simulink model "Appl_HeatAdj_CtrlModel"  (R2018b)
settings: configuration reference "CodeConfig_10_ms" (kept outside this file)
undefined symbols (not defined in the file): CAL_LEVEL3_TIMEOUT, CAL_SW_20min_TIMEOUT, D_1stLevel_36, D_2ndLevel_39, D_3rdLevel_45, D_3rdLevel_48, D_DRVHEAT_PID_D, D_DRVHEAT_PID_I, D_DRVHEAT_PID_P, D_HEAT_HEAT_DEF, D_SwsLevel_Temp, FALSE, TRUE
libraries: DareLib x111, simulink x1
(part 5 of 6)

== stateflow chart Appl_HeatAdj_CtrlModel/LogicCtrl/LocalAdjustCtrl/OutputDeal/HeatOutFunction2/HeatOut ==
  state PwmCnt = PidGetPwm(CurrentTemp,SetTemp) [function]
  state Controll [parallel]
    settings: executionOrder=1
    state AllOut
      en:
      du:
      HeatOutGpio = ON;
      HeatOutPwmCnt =100;
      TimeCnt = 0;
    state None
      en:
      du:
      HeatOutGpio = OFF;
      HeatOutPwmCnt = 0;
      TimeCnt = 0;
    state PwmOut
      en:
      HeatOutPwmCnt = PidGetPwm(CurrentTemp,SetTemp);
      (default) -> (junction 11)
      PwmOut -> (junction 11) [order 1]
      (junction 11) -> (junction 12) [order 1] : /* 100计数 */
          | [TimeCnt <= 100]
      (junction 11) -> (junction 15) [order 2] : /* 计算pid 算pwm */
          | {TimeCnt = 0;
          | HeatOutPwmCnt = PidGetPwm(CurrentTemp,SetTemp);}
      (junction 12) -> (junction 13) : {TimeCnt += 1;}
      (junction 13) -> (junction 14) [order 1] : [TimeCnt <= HeatOutPwmCnt]
      (junction 13) -> (junction 16) [order 2] : /* 引脚拉低 */
          | {HeatOutGpio = OFF;}
      (junction 14) -> (junction 17) : /* 引脚拉高 */
          | {HeatOutGpio = ON;}
      (junction 16) -> (junction 15)
      (junction 17) -> (junction 16)
      (junction 15) -> (junction 18)
    (default) -> None
    None -> AllOut [order 1] : /* 加热误差在3度 全开 */
        | [enHeatLvlSts.EN_HEAT_LVL_OFF < HeatLvl ...
        | && SetTemp > CurrentTemp ...
        | && (SetTemp - CurrentTemp) >= D_HEAT_HEAT_DEF]
    AllOut -> None [order 1] : /*全开 进 关 */
        | [SetTemp <= CurrentTemp ...
        | || enHeatLvlSts.EN_HEAT_LVL_OFF == HeatLvl]
    PwmOut -> None [order 1] : /* PID 进 关 */
        | [SetTemp <= CurrentTemp ...
        | || enHeatLvlSts.EN_HEAT_LVL_OFF == HeatLvl]
    None -> PwmOut [order 2] : /* 关 进 PID */
        | [enHeatLvlSts.EN_HEAT_LVL_OFF < HeatLvl ...
        | && SetTemp > CurrentTemp ...
        | && (SetTemp - CurrentTemp) < D_HEAT_HEAT_DEF]
    PwmOut -> AllOut [order 2] : /* 加热误差在3度 全开 */
        | [enHeatLvlSts.EN_HEAT_LVL_OFF < HeatLvl ...
        | && SetTemp > CurrentTemp ...
        | && (SetTemp - CurrentTemp) >= D_HEAT_HEAT_DEF]
    AllOut -> PwmOut [order 2] : /* 全开 进PID */
        | [enHeatLvlSts.EN_HEAT_LVL_OFF < HeatLvl ...
        | && SetTemp > CurrentTemp ...
        | && (SetTemp - CurrentTemp) < D_HEAT_HEAT_DEF]
  state count [parallel]
    settings: executionOrder=2
    (default) -> (junction 47)
    count -> (junction 47)
    (junction 47) -> (junction 50) [order 1] : /*方向盘加热开启且加热温度≥目标温度*/
        | [enHeatLvlSts.EN_HEAT_LVL_OFF < HeatLvl ...
        | && CurrentTemp >= (SetTemp - 20)]
    (junction 47) -> (junction 52) [order 2] : {Sw20minTimer = D_HAL_GET_CUR_MS_TS();}
    (junction 50) -> (junction 54)
    (junction 54) -> (junction 58) [order 1] : [TimeDiffTs(Sw20minTimer,D_HAL_GET_CUR_MS_TS()) < MaxTime]
    (junction 54) -> (junction 62) [order 2] : {SwTimeoutFlag = TRUE;}
    (junction 58) -> (junction 60) : {SwTimeoutFlag = FALSE;}
    (junction 62) -> (junction 52)
    (junction 60) -> (junction 62)
    (junction 52) -> (junction 66)
    (junction 66) -> (junction 82) [order 1] : [enHeatLvlSts.EN_HEAT_LVL_OFF == HeatLvl]
    (junction 66) -> (junction 87) [order 2]
    (junction 82) -> (junction 84) : {SwTimeoutFlag = FALSE;}
    (junction 84) -> (junction 87)
    (junction 87) -> (junction 92)
  state Ts = D_HAL_GET_CUR_MS_TS [function]
  state OutTs = TimeDiffTs(lastTs,Ts) [function]
  state count1 [parallel] [commented out]
    (default) -> (junction 103) [commented out]
    count1 -> (junction 103) [commented out]
    (junction 103) -> (junction 105) [commented out] : /*方向盘加热开启且加热温度≥目标温度*/
        | [enHeatLvlSts.EN_HEAT_LVL_OFF < HeatLvl ...
        | && CurrentTemp >= (SetTemp - 20)]
    (junction 103) -> (junction 111) [commented out]
    (junction 105) -> (junction 106) [commented out]
    (junction 106) -> (junction 108) [commented out] : [MaxTime > Sw20minTimer]
    (junction 106) -> (junction 107) [commented out] : {Sw20minTimer = MaxTime;
        | SwTimeoutFlag = TRUE;}
    (junction 108) -> (junction 113) [commented out] : {Sw20minTimer ++;
        | SwTimeoutFlag = FALSE;}
    (junction 107) -> (junction 111) [commented out]
    (junction 113) -> (junction 107) [commented out]
    (junction 111) -> (junction 114) [commented out]
    (junction 114) -> (junction 118) [commented out] : [enHeatLvlSts.EN_HEAT_LVL_OFF == HeatLvl]
    (junction 114) -> (junction 120) [commented out]
    (junction 118) -> (junction 102) [commented out] : {Sw20minTimer = 0;
        | SwTimeoutFlag = FALSE;}
    (junction 102) -> (junction 120) [commented out]
    (junction 120) -> (junction 101) [commented out]
  data: CurrentTemp function_input; PwmCnt function_output; SetTemp function_input; Ts function_output; lastTs function_input; Ts function_input; OutTs function_output; CurrentTemp input uint16; HeatLvl input Enum: enHeatLvlSts; SetTemp input uint16; HeatOutGpio output uint8; TimeCnt local uint8; OFF parameter; ON parameter; D_HEAT_HEAT_DEF parameter; HeatOutPwmCnt output uint8; TRUE parameter; FALSE parameter; SwTimeoutFlag output uint8 =0; Sw20minTimer output uint32; MaxTime input

== stateflow chart Appl_HeatAdj_CtrlModel/LogicCtrl/LocalAdjustCtrl/OutputDeal/HeatOutFunction2/HeatOut/PidGetPwm/Pid  ==
  (default) -> (junction 14)
  (junction 14) -> (junction 16) : /* 局部初始化 */
      | {Error = 0;
      | dError = 0;}
  (junction 16) -> (junction 20) : /* PID 计算 */
      | {Error = SetTemp - CurrentTemp;
      | SumError += Error;
      | dError = Error - LastError;
      | LastError = Error;
      | PwmCnt = (D_DRVHEAT_PID_P * Error)  + (D_DRVHEAT_PID_I *SumError) + (D_DRVHEAT_PID_D *  dError);}
  (junction 20) -> (junction 29) [order 1] : [PwmCnt > 100]
  (junction 20) -> (junction 27) [order 2]
  (junction 29) -> (junction 31) : {PwmCnt = 100;}
  (junction 31) -> (junction 27)
  (junction 27) -> (junction 34)
  data: dError local uint32; Error local uint32; CurrentTemp input uint16; SetTemp input uint16; PwmCnt output uint16; SumError local uint32; LastError local uint32; D_DRVHEAT_PID_P parameter; D_DRVHEAT_PID_I parameter; D_DRVHEAT_PID_D parameter

== stateflow chart Appl_HeatAdj_CtrlModel/LogicCtrl/LocalAdjustCtrl/LimitDeal/TimeoutFunction/Timeout ==
  state Ts = D_HAL_GET_CUR_MS_TS [function]
  state OutTs = TimeDiffTs(lastTs,Ts) [function]
  state TimeCountStatus
    state TimeoutSts
      en:
      Level = enHeatLvlSts.EN_HEAT_LVL_OFF;
      du:
      Level = enHeatLvlSts.EN_HEAT_LVL_OFF;
      ex:
      Timer = 0;
    state Init
      en:
      Level = InLevel;
      Timer = D_HAL_GET_CUR_MS_TS();
      du:
      Level = InLevel;
      ex:
      Timer = D_HAL_GET_CUR_MS_TS();
    (default) -> Init
    Init -> TimeoutSts [order 1] : [TimeDiffTs(Timer,D_HAL_GET_CUR_MS_TS()) >= MaxTime]
        | /TimeoutFlag = TRUE;
    TimeoutSts -> Init : [hasChangedFrom(InLevel,enHeatLvlSts.EN_HEAT_LVL_OFF)]
    Init -> Init [order 2] : [hasChangedFrom(InLevel,enHeatLvlSts.EN_HEAT_LVL_OFF)]
  state Default
    en:
    Level = InLevel;
    du:
    Level = InLevel;
  (default) -> Default
  Default -> TimeCountStatus : /*有超时配置
      | && 启动加热&&有时间值 */
      | [TRUE == TimeoutPrm ...
      | && enHeatLvlSts.EN_HEAT_LVL_OFF != InLevel ...
      | && 0 != MaxTime]
  TimeCountStatus -> Default : /*无超时配置*/
      | [TRUE != TimeoutPrm || 0 == MaxTime]
      | /TimeoutFlag = FALSE;
  data: Ts function_output; lastTs function_input; Ts function_input; OutTs function_output; TimeoutPrm input uint8; TimeoutFlag output uint8; FALSE parameter; TRUE parameter; InLevel input Enum: enHeatLvlSts; MaxTime input uint32; Timer local uint32; Level output Enum: enHeatLvlSts

== stateflow chart Appl_HeatAdj_CtrlModel/LogicCtrl/LocalAdjustCtrl/LimitDeal/TimeoutFunction/Timeout/TimeDiffTs/Chart ==
  (default) -> (junction 3)
  (junction 3) -> (junction 5)
  (junction 5) -> (junction 7) [order 1] : /* 入参比当前大 */
      | [lastTs > Ts]
  (junction 5) -> (junction 13) [order 2] : {OutTs = Ts - lastTs;}
  (junction 7) -> (junction 11) : {OutTs = 0xFFFFFFFF - lastTs + Ts +1;}
  (junction 11) -> (junction 13)
  (junction 13) -> (junction 17)
  data: lastTs input uint32; Ts input uint32; OutTs output uint32

== stateflow chart Appl_HeatAdj_CtrlModel/LogicCtrl/LocalAdjustCtrl/HeatLevelDeal/LevelAquireFunction2/LevelAquireFunction ==
  state LevelAquire
    (default) -> (junction 103)
    LevelAquire -> (junction 103)
    (junction 103) -> (junction 105) [order 1] : /*加热功能禁能
        | || 通用前置条件不满足)*/
        | [enHeatStopReason.EN_HEAT_STOP_R_NONE != DisableSts ...
        | || FALSE == EnableCfg ...
        | || TRUE != ComPCFlag]
    (junction 103) -> (junction 102) [order 2] : {StopFlag = FALSE;}
    (junction 105) -> (junction 104) : {Level = enHeatLvlSts.EN_HEAT_LVL_OFF;
        | StopFlag = TRUE;}
    (junction 104) -> (junction 102)
    (junction 102) -> (junction 111)
    (junction 111) -> (junction 21) [order 1] : [FALSE == StopFlag]
    (junction 21) -> (junction 23) [order 1] : [enProjectType.EN_PROJECT_P20 == CarTypeCfg]
    (junction 111) -> (junction 114) [order 2] : {Level = enHeatLvlSts.EN_HEAT_LVL_OFF;}
    (junction 21) -> (junction 48) [order 2]
    (junction 23) -> (junction 85)
    (junction 85) -> (junction 87) [order 1] : /* open 信号 且为HMI控制*/
        | [5 == CAN_Message && Type == FALSE]
    (junction 85) -> (junction 25) [order 2]
    (junction 87) -> (junction 89) : {Level = CanLvl + 1;}
    (junction 25) -> (junction 27) [order 1] : [4 == CAN_Message]
    (junction 25) -> (junction 29) [order 2] : {TempMsg = CAN_Message + 1;}
    (junction 27) -> (junction 57) : {Level = enHeatLvlSts.EN_HEAT_LVL_OFF;}
    (junction 48) -> (junction 50) [order 1] : [1 != CAN_Message]
    (junction 48) -> (junction 55) [order 2] : {Level = enHeatLvlSts.EN_HEAT_LVL_OFF;}
    (junction 50) -> (junction 52) : {TempMsg = CAN_Message;}
    (junction 52) -> (junction 29)
    (junction 29) -> (junction 32) [order 1] : [1 < TempMsg && 5 > TempMsg]
    (junction 29) -> (junction 36) [order 2] : {Level = 0xFF;}
    (junction 32) -> (junction 34)
    (junction 34) -> (junction 38) [order 1] : [2 == TempMsg]
    (junction 34) -> (junction 40) [order 2]
    (junction 38) -> (junction 59) : {Level = enHeatLvlSts.EN_HEAT_LVL_1;}
    (junction 40) -> (junction 42) [order 1] : [3 == TempMsg]
    (junction 40) -> (junction 46) [order 2] : {Level = enHeatLvlSts.EN_HEAT_LVL_3;}
    (junction 42) -> (junction 44) : {Level = enHeatLvlSts.EN_HEAT_LVL_2;}
    (junction 55) -> (junction 114)
    (junction 36) -> (junction 55)
    (junction 46) -> (junction 36)
    (junction 44) -> (junction 46)
    (junction 59) -> (junction 44)
    (junction 57) -> (junction 59)
    (junction 89) -> (junction 57)
    (junction 114) -> (junction 75)
  data: EnableCfg input uint8; CarTypeCfg input Enum: enProjectType; CAN_Message input uint8; DisableSts input Enum: enHeatStopReason; Level output uint8; TempMsg local uint8; TRUE parameter; FALSE parameter; ComPCFlag input; CanLvl input uint8; Type input; CurLvl input; StopFlag local boolean

== stateflow chart Appl_HeatAdj_CtrlModel/UpDataInputInfo/InputSignalProcess/HeatMessage/HeatMessage ==
  state [OutMsgHMI,OutMsgTbox,MixConflictFlg] = MsgConflictFunction2(CarTypeCfg,HMI_Message,Tbox_Message,VentValidFlag) [function]
  state [OutMsgHMI,OutMsgTbox,MixConflictFlg] = MsgConflictFunction1(CarTypeCfg,HMI_Message,Tbox_Message,VentValidFlag) [function]
  state [OutMsgHMI,OutMsgTbox,MixConflictFlg] = MsgConflictFunction(CarTypeCfg,HMI_Message,Tbox_Message,VentValidFlag) [function]
  state Message
    du:
    [DriverHMI_Message,DriverTbox_Message,Driver_MixConflicFlg] = MsgConflictFunction(HeatAdj_CarType,HeatAdj_DriverHMI_Message,HeatAdj_DriverTbox_Message,DriverVentilateValid);
    [PassengerHMI_Message,PassengerTbox_Message,Passenger_MixConflicFlg] = MsgConflictFunction1(HeatAdj_CarType,HeatAdj_PassengerHMI_Message,HeatAdj_PassengerTbox_Message,PassengerVentilateValid);
    [ThirdHMI_Message,ThirdTbox_Message,Third_MixConflicFlg] = MsgConflictFunction2(HeatAdj_CarType,HeatAdj_ThirdHMI_Message,HeatAdj_ThirdTbox_Message,ThirdVentilateValid);
  (default) -> Message
  data: CarTypeCfg function_input; HMI_Message function_input uint8; Tbox_Message function_input uint8; VentValidFlag function_input; OutMsgHMI function_output; OutMsgTbox function_output; MixConflictFlg function_output; CarTypeCfg function_input; HMI_Message function_input uint8; Tbox_Message function_input uint8; VentValidFlag function_input; OutMsgHMI function_output; OutMsgTbox function_output; MixConflictFlg function_output; CarTypeCfg function_input; HMI_Message function_input uint8; Tbox_Message function_input uint8; VentValidFlag function_input; OutMsgHMI function_output; OutMsgTbox function_output; MixConflictFlg function_output; DriverHMI_Message output uint8; DriverTbox_Message output uint8; PassengerHMI_Message output uint8; HeatAdj_DriverHMI_Message input; HeatAdj_DriverTbox_Message input; HeatAdj_PassengerHMI_Message input; HeatAdj_PassengerTbox_Message input; HeatAdj_ThirdHMI_Message input; HeatAdj_ThirdTbox_Message input; DriverVentilateValid input; PassengerVentilateValid input; ThirdVentilateValid input; PassengerTbox_Message output uint8; ThirdHMI_Message output uint8; ThirdTbox_Message output uint8; HeatAdj_CarType input; Driver_MixConflicFlg output uint8; Passenger_MixConflicFlg output uint8; Third_MixConflicFlg output uint8

== stateflow chart Appl_HeatAdj_CtrlModel/UpDataInputInfo/InputSignalProcess/HeatMessage/HeatMessage/MsgConflictFunction/Function ==
  state HMI_MessageDeal [parallel]
    settings: executionOrder=1
    state Default
      en:
      HMI_Flag = FALSE;
    state Valid
      en:
      HMI_Flag = TRUE;
    (default) -> HMI_MessageDeal.Default
    HMI_MessageDeal.Default -> HMI_MessageDeal.Valid : /*HMI加热报文有效0x0:Inactive；0x1:Level 1；1档;0x2:Level 2；2档;0x3:Level 3；3档；0x4:OFF: 0x05 OPEN*/
        | [enHeatLvlSts.EN_HEAT_LVL_1 == HMI_Message ...
        | || enHeatLvlSts.EN_HEAT_LVL_2 == HMI_Message ...
        | || enHeatLvlSts.EN_HEAT_LVL_3 == HMI_Message ...
        | || 4 == HMI_Message || 5 == HMI_Message]
    HMI_MessageDeal.Valid -> HMI_MessageDeal.Default : /*HMI加热报文无效，20240507NXM增加关闭4*/
        | [enHeatLvlSts.EN_HEAT_LVL_1 != HMI_Message ...
        | && enHeatLvlSts.EN_HEAT_LVL_2 != HMI_Message ...
        | && enHeatLvlSts.EN_HEAT_LVL_3 != HMI_Message ...
        | && 4 != HMI_Message && 5 != HMI_Message]
  state Tbox_MessageDeal [parallel]
    settings: executionOrder=2
    state Default
      en:
      Tbox_Flag = FALSE;
    state Valid
      en:
      Tbox_Flag = TRUE;
    (default) -> Tbox_MessageDeal.Default
    Tbox_MessageDeal.Default -> Tbox_MessageDeal.Valid : /*Tbox加热报文有效0x0:No Request；0x1:Heat_1；0x2:Heat_2；0x3:Heat_3；0x4:Close*/
        | [enHeatLvlSts.EN_HEAT_LVL_1 == Tbox_Message ...
        | || enHeatLvlSts.EN_HEAT_LVL_2 == Tbox_Message ...
        | || enHeatLvlSts.EN_HEAT_LVL_3 == Tbox_Message ...
        | || 4 == Tbox_Message]
    Tbox_MessageDeal.Valid -> Tbox_MessageDeal.Default : /*Tbox加热报文无效，20240507NXM增加关闭4*/
        | [enHeatLvlSts.EN_HEAT_LVL_1 != Tbox_Message ...
        | && enHeatLvlSts.EN_HEAT_LVL_2 != Tbox_Message ...
        | && enHeatLvlSts.EN_HEAT_LVL_3 != Tbox_Message ...
        | && 4 != Tbox_Message]
  state MessageConflictDeal [parallel]
    settings: executionOrder=3
    state Default
      en,du:
      OutMsgHMI = HMI_Message;
      OutMsgTbox = Tbox_Message;
      MixConflictFlg = FALSE;
    state VentilateConflict
      en:
      OutMsgHMI = 0;
      OutMsgTbox = 0;
      MixConflictFlg = TRUE;
    state HeatConflict
      en:
      OutMsgHMI = 0;
      OutMsgTbox = 0;
      MixConflictFlg = FALSE;
    (default) -> MessageConflictDeal.Default
    MessageConflictDeal.Default -> VentilateConflict [order 2] : /*通风加热报文同时有效 不包含关闭 */
        | [FALSE != VentValidFlag ...
        | && ((FALSE != HMI_Flag && 4 != HMI_Message)...
        | || (FALSE != Tbox_Flag && 4 != Tbox_Message))]
    VentilateConflict -> MessageConflictDeal.Default [order 2] : /*通风加热报文不同时有效或关闭，20240507NXM修改跳转顺序*/
        | [FALSE == VentValidFlag ...
        | || 4 == HMI_Message ...
        | || 4 == Tbox_Message]
    MessageConflictDeal.Default -> HeatConflict [order 1] : /*P20车型HMI、TBOX加热报文同时有效*/
        | [enProjectType.EN_PROJECT_P20 == CarTypeCfg ...
        | && FALSE != HMI_Flag ...
        | && FALSE != Tbox_Flag]
    HeatConflict -> MessageConflictDeal.Default [order 2] : /*非P20车型||P20车型加热报文不同时有效，20240507NXM*/
        | [enProjectType.EN_PROJECT_P20 != CarTypeCfg ...
        | || (enProjectType.EN_PROJECT_P20 == CarTypeCfg ...
        | && (FALSE == HMI_Flag || FALSE == Tbox_Flag))]
    VentilateConflict -> HeatConflict [order 1] : /*P20车型HMI、TBOX加热报文同时有效*/
        | [enProjectType.EN_PROJECT_P20 == CarTypeCfg ...
        | && FALSE != HMI_Flag ...
        | && FALSE != Tbox_Flag ...
        | && FALSE == VentValidFlag]
    HeatConflict -> VentilateConflict [order 1] : /*通风加热报文同时有效，20240507NXM*/
        | [FALSE != VentValidFlag ...
        | && (FALSE != HMI_Flag ...
        | || FALSE != Tbox_Flag)]
  data: CarTypeCfg input uint8; HMI_Message input; Tbox_Message input; VentValidFlag input uint8; FALSE parameter; OutMsgHMI output uint8; OutMsgTbox output uint8; HMI_Flag local uint8; Tbox_Flag local uint8; TRUE parameter; MixConflictFlg output uint8

== stateflow chart Appl_HeatAdj_CtrlModel/UpDataInputInfo/InputSignalProcess/CommonPreconditionDeal/Deal ==
  state Default
    en:
    ComPCSatisfiedFlag = FALSE;
  state ValidSts
    en:
    ComPCSatisfiedFlag = TRUE;
  (default) -> Default
  Default -> ValidSts : /*非OFF电 && DCDC开关状态为使能
      | && 正常电压模式下
      | && (发动机运行中 || 整车运行状态满足)*/
      | [enPowerModeSts.EN_OFF != HeatAdj_PowerMode ...
      | && TRUE == DCDC_SwitchEnable ...
      | && enFinalPowerMode.EN_NORMAL_VOLT == HeatAdj_VoltMode ...
      | && (TRUE == EngineRunningFlag || TRUE == VehicleRunFlag)]
  ValidSts -> Default : /*OFF电 || DCDC开关状态为非使能 || 非正常电压
      | || (发动机不在运行中 && 整车运行状态不满足)*/
      | [enPowerModeSts.EN_OFF == HeatAdj_PowerMode ...
      | || TRUE != DCDC_SwitchEnable ...
      | || enFinalPowerMode.EN_NORMAL_VOLT != HeatAdj_VoltMode ...
      | || (TRUE != EngineRunningFlag && TRUE != VehicleRunFlag)]
  data: HeatAdj_PowerMode input; DCDC_SwitchEnable input; EngineRunningFlag input; VehicleRunFlag input; ComPCSatisfiedFlag output uint8; TRUE parameter; FALSE parameter; HeatAdj_VoltMode input

== stateflow chart Appl_HeatAdj_CtrlModel/LogicCtrl/LocalAdjustCtrl/HeatLevelDeal/LevelAquireFunction4/LevelAquireFunction ==
  state LevelAquire
    (default) -> (junction 103)
    LevelAquire -> (junction 103)
    (junction 103) -> (junction 105) [order 1] : /*加热功能禁能
        | || 通用前置条件不满足)*/
        | [enHeatStopReason.EN_HEAT_STOP_R_NONE != DisableSts ...
        | || FALSE == EnableCfg ...
        | || TRUE != ComPCFlag]
    (junction 103) -> (junction 102) [order 2] : {StopFlag = FALSE;}
    (junction 105) -> (junction 104) : {Level = enHeatLvlSts.EN_HEAT_LVL_OFF;
        | StopFlag = TRUE;}
    (junction 104) -> (junction 102)
    (junction 102) -> (junction 111)
    (junction 111) -> (junction 21) [order 1] : [FALSE == StopFlag]
    (junction 21) -> (junction 23) [order 1] : [enProjectType.EN_PROJECT_P20 == CarTypeCfg]
    (junction 111) -> (junction 114) [order 2] : {Level = enHeatLvlSts.EN_HEAT_LVL_OFF;}
    (junction 21) -> (junction 48) [order 2]
    (junction 23) -> (junction 85)
    (junction 85) -> (junction 87) [order 1] : /* open 信号 且为HMI控制*/
        | [5 == CAN_Message && Type == FALSE]
    (junction 85) -> (junction 25) [order 2]
    (junction 87) -> (junction 89) : {Level = CanLvl + 1;}
    (junction 25) -> (junction 27) [order 1] : [4 == CAN_Message]
    (junction 25) -> (junction 29) [order 2] : {TempMsg = CAN_Message + 1;}
    (junction 27) -> (junction 57) : {Level = enHeatLvlSts.EN_HEAT_LVL_OFF;}
    (junction 48) -> (junction 50) [order 1] : [1 != CAN_Message]
    (junction 48) -> (junction 55) [order 2] : {Level = enHeatLvlSts.EN_HEAT_LVL_OFF;}
    (junction 50) -> (junction 52) : {TempMsg = CAN_Message;}
    (junction 52) -> (junction 29)
    (junction 29) -> (junction 32) [order 1] : [1 < TempMsg && 5 > TempMsg]
    (junction 29) -> (junction 36) [order 2] : {Level = 0xFF;}
    (junction 32) -> (junction 34)
    (junction 34) -> (junction 38) [order 1] : [2 == TempMsg]
    (junction 34) -> (junction 40) [order 2]
    (junction 38) -> (junction 59) : {Level = enHeatLvlSts.EN_HEAT_LVL_1;}
    (junction 40) -> (junction 42) [order 1] : [3 == TempMsg]
    (junction 40) -> (junction 46) [order 2] : {Level = enHeatLvlSts.EN_HEAT_LVL_3;}
    (junction 42) -> (junction 44) : {Level = enHeatLvlSts.EN_HEAT_LVL_2;}
    (junction 55) -> (junction 114)
    (junction 36) -> (junction 55)
    (junction 46) -> (junction 36)
    (junction 44) -> (junction 46)
    (junction 59) -> (junction 44)
    (junction 57) -> (junction 59)
    (junction 89) -> (junction 57)
    (junction 114) -> (junction 75)
  data: EnableCfg input uint8; CarTypeCfg input Enum: enProjectType; CAN_Message input uint8; DisableSts input Enum: enHeatStopReason; Level output uint8; TempMsg local uint8; TRUE parameter; FALSE parameter; ComPCFlag input; CanLvl input uint8; Type input; CurLvl input; StopFlag local boolean

== stateflow chart Appl_HeatAdj_CtrlModel/LogicCtrl/LocalAdjustCtrl/HeatLevelDeal/LevelAquireFunction/LevelAquireFunction ==
  state LevelAquire
    (default) -> (junction 103)
    LevelAquire -> (junction 103)
    (junction 103) -> (junction 105) [order 1] : /*加热功能禁能
        | || 通用前置条件不满足)*/
        | [enHeatStopReason.EN_HEAT_STOP_R_NONE != DisableSts ...
        | || FALSE == EnableCfg ...
        | || TRUE != ComPCFlag]
    (junction 103) -> (junction 102) [order 2] : {StopFlag = FALSE;}
    (junction 105) -> (junction 104) : {Level = enHeatLvlSts.EN_HEAT_LVL_OFF;
        | StopFlag = TRUE;}
    (junction 104) -> (junction 102)
    (junction 102) -> (junction 111)
    (junction 111) -> (junction 21) [order 1] : [FALSE == StopFlag]
    (junction 21) -> (junction 23) [order 1] : [enProjectType.EN_PROJECT_P20 == CarTypeCfg]
    (junction 111) -> (junction 114) [order 2] : {Level = enHeatLvlSts.EN_HEAT_LVL_OFF;}
    (junction 21) -> (junction 48) [order 2]
    (junction 23) -> (junction 85)
    (junction 85) -> (junction 87) [order 1] : /* open 信号 且为HMI控制*/
        | [5 == CAN_Message && Type == FALSE]
    (junction 85) -> (junction 25) [order 2]
    (junction 87) -> (junction 89) : {Level = CanLvl + 1;}
    (junction 25) -> (junction 27) [order 1] : [4 == CAN_Message]
    (junction 25) -> (junction 29) [order 2] : {TempMsg = CAN_Message + 1;}
    (junction 27) -> (junction 57) : {Level = enHeatLvlSts.EN_HEAT_LVL_OFF;}
    (junction 48) -> (junction 50) [order 1] : [1 != CAN_Message]
    (junction 48) -> (junction 55) [order 2] : {Level = enHeatLvlSts.EN_HEAT_LVL_OFF;}
    (junction 50) -> (junction 52) : {TempMsg = CAN_Message;}
    (junction 52) -> (junction 29)
    (junction 29) -> (junction 32) [order 1] : [1 < TempMsg && 5 > TempMsg]
    (junction 29) -> (junction 36) [order 2] : {Level = 0xFF;}
    (junction 32) -> (junction 34)
    (junction 34) -> (junction 38) [order 1] : [2 == TempMsg]
    (junction 34) -> (junction 40) [order 2]
    (junction 38) -> (junction 59) : {Level = enHeatLvlSts.EN_HEAT_LVL_1;}
    (junction 40) -> (junction 42) [order 1] : [3 == TempMsg]
    (junction 40) -> (junction 46) [order 2] : {Level = enHeatLvlSts.EN_HEAT_LVL_3;}
    (junction 42) -> (junction 44) : {Level = enHeatLvlSts.EN_HEAT_LVL_2;}
    (junction 55) -> (junction 114)
    (junction 36) -> (junction 55)
    (junction 46) -> (junction 36)
    (junction 44) -> (junction 46)
    (junction 59) -> (junction 44)
    (junction 57) -> (junction 59)
    (junction 89) -> (junction 57)
    (junction 114) -> (junction 75)
  data: EnableCfg input uint8; CarTypeCfg input Enum: enProjectType; CAN_Message input uint8; DisableSts input Enum: enHeatStopReason; Level output uint8; TempMsg local uint8; TRUE parameter; FALSE parameter; ComPCFlag input; CanLvl input uint8; Type input; CurLvl input; StopFlag local boolean

== stateflow chart Appl_HeatAdj_CtrlModel/LogicCtrl/LocalAdjustCtrl/HeatLevelDeal/LevelAquireFunction5/LevelAquireFunction ==
  state LevelAquire
    (default) -> (junction 103)
    LevelAquire -> (junction 103)
    (junction 103) -> (junction 105) [order 1] : /*加热功能禁能
        | || 通用前置条件不满足)*/
        | [enHeatStopReason.EN_HEAT_STOP_R_NONE != DisableSts ...
        | || FALSE == EnableCfg ...
        | || TRUE != ComPCFlag]
    (junction 103) -> (junction 102) [order 2] : {StopFlag = FALSE;}
    (junction 105) -> (junction 104) : {Level = enHeatLvlSts.EN_HEAT_LVL_OFF;
        | StopFlag = TRUE;}
    (junction 104) -> (junction 102)
    (junction 102) -> (junction 111)
    (junction 111) -> (junction 21) [order 1] : [FALSE == StopFlag]
    (junction 21) -> (junction 23) [order 1] : [enProjectType.EN_PROJECT_P20 == CarTypeCfg]
    (junction 111) -> (junction 114) [order 2] : {Level = enHeatLvlSts.EN_HEAT_LVL_OFF;}
    (junction 21) -> (junction 48) [order 2]
    (junction 23) -> (junction 85)
    (junction 85) -> (junction 87) [order 1] : /* open 信号 且为HMI控制*/
        | [5 == CAN_Message && Type == FALSE]
    (junction 85) -> (junction 25) [order 2]
    (junction 87) -> (junction 89) : {Level = CanLvl + 1;}
    (junction 25) -> (junction 27) [order 1] : [4 == CAN_Message]
    (junction 25) -> (junction 29) [order 2] : {TempMsg = CAN_Message + 1;}
    (junction 27) -> (junction 57) : {Level = enHeatLvlSts.EN_HEAT_LVL_OFF;}
    (junction 48) -> (junction 50) [order 1] : [1 != CAN_Message]
    (junction 48) -> (junction 55) [order 2] : {Level = enHeatLvlSts.EN_HEAT_LVL_OFF;}
    (junction 50) -> (junction 52) : {TempMsg = CAN_Message;}
    (junction 52) -> (junction 29)
    (junction 29) -> (junction 32) [order 1] : [1 < TempMsg && 5 > TempMsg]
    (junction 29) -> (junction 36) [order 2] : {Level = 0xFF;}
    (junction 32) -> (junction 34)
    (junction 34) -> (junction 38) [order 1] : [2 == TempMsg]
    (junction 34) -> (junction 40) [order 2]
    (junction 38) -> (junction 59) : {Level = enHeatLvlSts.EN_HEAT_LVL_1;}
    (junction 40) -> (junction 42) [order 1] : [3 == TempMsg]
    (junction 40) -> (junction 46) [order 2] : {Level = enHeatLvlSts.EN_HEAT_LVL_3;}
    (junction 42) -> (junction 44) : {Level = enHeatLvlSts.EN_HEAT_LVL_2;}
    (junction 55) -> (junction 114)
    (junction 36) -> (junction 55)
    (junction 46) -> (junction 36)
    (junction 44) -> (junction 46)
    (junction 59) -> (junction 44)
    (junction 57) -> (junction 59)
    (junction 89) -> (junction 57)
    (junction 114) -> (junction 75)
  data: EnableCfg input uint8; CarTypeCfg input Enum: enProjectType; CAN_Message input uint8; DisableSts input Enum: enHeatStopReason; Level output uint8; TempMsg local uint8; TRUE parameter; FALSE parameter; ComPCFlag input; CanLvl input uint8; Type input; CurLvl input; StopFlag local boolean

== stateflow chart Appl_HeatAdj_CtrlModel/LogicCtrl/LocalAdjustCtrl/HeatLevelDeal/LevelAquireFunction3/LevelAquireFunction ==
  state LevelAquire
    (default) -> (junction 103)
    LevelAquire -> (junction 103)
    (junction 103) -> (junction 105) [order 1] : /*加热功能禁能
        | || 通用前置条件不满足)*/
        | [enHeatStopReason.EN_HEAT_STOP_R_NONE != DisableSts ...
        | || FALSE == EnableCfg ...
        | || TRUE != ComPCFlag]
    (junction 103) -> (junction 102) [order 2] : {StopFlag = FALSE;}
    (junction 105) -> (junction 104) : {Level = enHeatLvlSts.EN_HEAT_LVL_OFF;
        | StopFlag = TRUE;}
    (junction 104) -> (junction 102)
    (junction 102) -> (junction 111)
    (junction 111) -> (junction 21) [order 1] : [FALSE == StopFlag]
    (junction 21) -> (junction 23) [order 1] : [enProjectType.EN_PROJECT_P20 == CarTypeCfg]
    (junction 111) -> (junction 114) [order 2] : {Level = enHeatLvlSts.EN_HEAT_LVL_OFF;}
    (junction 21) -> (junction 48) [order 2]
    (junction 23) -> (junction 85)
    (junction 85) -> (junction 87) [order 1] : /* open 信号 且为HMI控制*/
        | [5 == CAN_Message && Type == FALSE]
    (junction 85) -> (junction 25) [order 2]
    (junction 87) -> (junction 89) : {Level = CanLvl + 1;}
    (junction 25) -> (junction 27) [order 1] : [4 == CAN_Message]
    (junction 25) -> (junction 29) [order 2] : {TempMsg = CAN_Message + 1;}
    (junction 27) -> (junction 57) : {Level = enHeatLvlSts.EN_HEAT_LVL_OFF;}
    (junction 48) -> (junction 50) [order 1] : [1 != CAN_Message]
    (junction 48) -> (junction 55) [order 2] : {Level = enHeatLvlSts.EN_HEAT_LVL_OFF;}
    (junction 50) -> (junction 52) : {TempMsg = CAN_Message;}
    (junction 52) -> (junction 29)
    (junction 29) -> (junction 32) [order 1] : [1 < TempMsg && 5 > TempMsg]
    (junction 29) -> (junction 36) [order 2] : {Level = 0xFF;}
    (junction 32) -> (junction 34)
    (junction 34) -> (junction 38) [order 1] : [2 == TempMsg]
    (junction 34) -> (junction 40) [order 2]
    (junction 38) -> (junction 59) : {Level = enHeatLvlSts.EN_HEAT_LVL_1;}
    (junction 40) -> (junction 42) [order 1] : [3 == TempMsg]
    (junction 40) -> (junction 46) [order 2] : {Level = enHeatLvlSts.EN_HEAT_LVL_3;}
    (junction 42) -> (junction 44) : {Level = enHeatLvlSts.EN_HEAT_LVL_2;}
    (junction 55) -> (junction 114)
    (junction 36) -> (junction 55)
    (junction 46) -> (junction 36)
    (junction 44) -> (junction 46)
    (junction 59) -> (junction 44)
    (junction 57) -> (junction 59)
    (junction 89) -> (junction 57)
    (junction 114) -> (junction 75)
  data: EnableCfg input uint8; CarTypeCfg input Enum: enProjectType; CAN_Message input uint8; DisableSts input Enum: enHeatStopReason; Level output uint8; TempMsg local uint8; TRUE parameter; FALSE parameter; ComPCFlag input; CanLvl input uint8; Type input; CurLvl input; StopFlag local boolean

== stateflow chart Appl_HeatAdj_CtrlModel/UpDataInputInfo/InputSignalProcess/VehRunSta/VehicleRunStatus ==
  state Default
    en:
    VehicleRunFlag = FALSE;
  state ValidSts
    en:
    VehicleRunFlag = TRUE;
  (default) -> Default
  Default -> ValidSts : /*（平台发动机配置字使能
      | && P20车型配置字使能
      | && VCU_VehRunSta= 0x1:HV ON /0x2:Ready）
      | || 平台发动机配置字禁能
      | || 非P20车型*/
      | [(TRUE == HeatAdj_PlatformVehicleEnableConfig ...
      | && TRUE == HeatAdj_P20_PHEV_EngineCfg ...
      | && (enVehicleRunType.EN_HV_ON == HeatAdj_VCU_VehRunSta ...
      | || enVehicleRunType.EN_HV_READY == HeatAdj_VCU_VehRunSta)) ...
      | || FALSE == HeatAdj_PlatformVehicleEnableConfig ...
      | || enProjectType.EN_PROJECT_P20 != HeatAdj_CarType]
  ValidSts -> Default : /*平台整车配置字使能
      | && P20车型配置字使能
      | && V整车运行状态非0x1:HV ON /0x2:Ready(0x3:Invalid保持上一状态)*/
      | [TRUE == HeatAdj_PlatformVehicleEnableConfig ...
      | && (TRUE != HeatAdj_P20_PHEV_EngineCfg ...
      | || enVehicleRunType.EN_HV_OFF == HeatAdj_VCU_VehRunSta)]
  data: FALSE parameter; TRUE parameter; VehicleRunFlag output uint8; HeatAdj_PlatformVehicleEnableConfig input; HeatAdj_P20_PHEV_EngineCfg input; HeatAdj_VCU_VehRunSta input; HeatAdj_CarType input

== stateflow chart Appl_HeatAdj_CtrlModel/LogicCtrl/LocalAdjustCtrl/HeatLevelDeal/CANAquireFunction/CANAquireFunction ==
  state HeatDisable
    en:
    IVISwCan = enSteerHeatType.EN_STEER_NONE;
    TempMsg = 0;
  state ValidSts
    ex:
    TempMsg = 0;
    ValidCnt = 0;
    (default) -> (junction 85)
    ValidSts -> (junction 85) [order 1]
    (junction 85) -> (junction 88) [order 1] : /*加热已通过其他方式开启*/
        | [enHeatLvlSts.EN_HEAT_LVL_OFF != HeatLevel ...
        | && enSteerHeatType.EN_STEER_OPEN != TempMsg]
    (junction 85) -> (junction 92) [order 2] : {IVISwCan = enSteerHeatType.EN_STEER_OPEN;
        | TempMsg = enSteerHeatType.EN_STEER_OPEN;}
    (junction 88) -> (junction 90) : {IVISwCan = enSteerHeatType.EN_STEER_NONE;}
    (junction 90) -> (junction 92)
    (junction 92) -> (junction 95)
    (junction 95) -> (junction 98) [order 1] : [ValidCnt < 3]
    (junction 95) -> (junction 102) [order 2] : {ValidCnt = 3;}
    (junction 98) -> (junction 100) : {ValidCnt ++;}
    (junction 100) -> (junction 102)
    (junction 102) -> (junction 105)
  state CloseSts
    en:
    IVISwCan = enSteerHeatType.EN_STEER_CLOSE;
  (default) -> HeatDisable
  HeatDisable -> ValidSts : /*(非OFF 电 && 加热未启动 && 开关变为有效)
      | || 加热已开启*/
      | [(enPowerModeSts.EN_OFF != PowerMode ...
      | && enHeatLvlSts.EN_HEAT_LVL_OFF == HeatLevel ...
      | && hasChangedTo(IVISwsHeat,1)) ...
      | || enHeatLvlSts.EN_HEAT_LVL_OFF != HeatLevel]
  ValidSts -> HeatDisable [order 2] : /*其他模式、故障关闭加热*/
      | [enHeatLvlSts.EN_HEAT_LVL_OFF == HeatLevel ...
      | && 3 == ValidCnt]
  CloseSts -> HeatDisable : /*IVI_SwsHeatSw = 0x0:Not Pressed
      | || 事件报文超时后（Event = 20ms）*/
      | [0 == IVISwsHeat ...
      | || after(5,tick)]
  ValidSts -> CloseSts [order 1] : /*(非OFF 电 && 加热已启动 && 开关变为有效)
      | || OFF电*/
      | [(enPowerModeSts.EN_OFF != PowerMode ...
      | && enHeatLvlSts.EN_HEAT_LVL_OFF != HeatLevel ...
      | && hasChangedTo(IVISwsHeat,1)) ...
      | || enPowerModeSts.EN_OFF == PowerMode]
  data: HeatLevel input uint8; IVISwsHeat input uint8; PowerMode input Enum: enPowerModeSts; IVISwCan output uint8; TempMsg local uint8; ValidCnt local uint8

== stateflow chart Appl_HeatAdj_CtrlModel/LogicCtrl/LocalAdjustCtrl/HeatLevelDeal/SwLevelAquireFunction/SwLevelAquireFunction ==
  state LevelAquire
    (default) -> (junction 181)
    LevelAquire -> (junction 181)
    (junction 181) -> (junction 177) [order 1] : /*存在禁能条件时，不再输出有效加热请求*/
        | /*加热功能禁能
        | || 通用前置条件不满足)*/
        | [enHeatStopReason.EN_HEAT_STOP_R_NONE != DisableSts ...
        | || FALSE == EnableCfg ...
        | || TRUE != ComPCFlag]
    (junction 181) -> (junction 184) [order 2] : {StopFlag = FALSE;}
    (junction 177) -> (junction 176) : {Level = enHeatLvlSts.EN_HEAT_LVL_OFF;
        | StopFlag = TRUE;}
    (junction 176) -> (junction 184)
    (junction 184) -> (junction 185)
    (junction 185) -> (junction 48) [order 1] : [FALSE == StopFlag]
    (junction 48) -> (junction 50) [order 1] : /*P20
        | 0x0:无动作
        | 0x1:开始
        | 0x2:关闭
        | 0x3:无效值*/
        | [0x02 == CAN_Message]
    (junction 185) -> (junction 188) [order 2] : {Level = enHeatLvlSts.EN_HEAT_LVL_OFF;}
    (junction 48) -> (junction 142) [order 2]
    (junction 50) -> (junction 52) : {Level = enHeatLvlSts.EN_HEAT_LVL_OFF;}
    (junction 142) -> (junction 144) [order 1] : /*P20
        | 0x0:无动作
        | 0x1:开始
        | 0x2:关闭
        | 0x3:无效值*/
        | [0x01 == CAN_Message]
    (junction 142) -> (junction 55) [order 2] : {Level = 0xFF;}
    (junction 144) -> (junction 146) : {Level = enHeatLvlSts.EN_HEAT_LVL_3;}
    (junction 55) -> (junction 188)
    (junction 146) -> (junction 55)
    (junction 52) -> (junction 146)
    (junction 188) -> (junction 75)
  data: EnableCfg input uint8; CAN_Message input uint8; DisableSts input Enum: enHeatStopReason; Level output uint8; TRUE parameter; FALSE parameter; ComPCFlag input; StopFlag local boolean

== stateflow chart Appl_HeatAdj_CtrlModel/UpDataInputInfo/InputSignalProcess/HeatMessage/HeatMessage/MsgConflictFunction1/Function ==
  state HMI_MessageDeal [parallel]
    settings: executionOrder=1
    state Default
      en:
      HMI_Flag = FALSE;
    state Valid
      en:
      HMI_Flag = TRUE;
    (default) -> HMI_MessageDeal.Default
    HMI_MessageDeal.Default -> HMI_MessageDeal.Valid : /*HMI加热报文有效0x0:Inactive；0x1:Level 1；1档;0x2:Level 2；2档;0x3:Level 3；3档；0x4:OFF: 0x05 OPEN*/
        | [enHeatLvlSts.EN_HEAT_LVL_1 == HMI_Message ...
        | || enHeatLvlSts.EN_HEAT_LVL_2 == HMI_Message ...
        | || enHeatLvlSts.EN_HEAT_LVL_3 == HMI_Message ...
        | || 4 == HMI_Message || 5 == HMI_Message]
    HMI_MessageDeal.Valid -> HMI_MessageDeal.Default : /*HMI加热报文无效，20240507NXM增加关闭4*/
        | [enHeatLvlSts.EN_HEAT_LVL_1 != HMI_Message ...
        | && enHeatLvlSts.EN_HEAT_LVL_2 != HMI_Message ...
        | && enHeatLvlSts.EN_HEAT_LVL_3 != HMI_Message ...
        | && 4 != HMI_Message && 5 != HMI_Message]
  state Tbox_MessageDeal [parallel]
    settings: executionOrder=2
    state Default
      en:
      Tbox_Flag = FALSE;
    state Valid
      en:
      Tbox_Flag = TRUE;
    (default) -> Tbox_MessageDeal.Default
    Tbox_MessageDeal.Default -> Tbox_MessageDeal.Valid : /*Tbox加热报文有效0x0:No Request；0x1:Heat_1；0x2:Heat_2；0x3:Heat_3；0x4:Close*/
        | [enHeatLvlSts.EN_HEAT_LVL_1 == Tbox_Message ...
        | || enHeatLvlSts.EN_HEAT_LVL_2 == Tbox_Message ...
        | || enHeatLvlSts.EN_HEAT_LVL_3 == Tbox_Message ...
        | || 4 == Tbox_Message]
    Tbox_MessageDeal.Valid -> Tbox_MessageDeal.Default : /*Tbox加热报文无效，20240507NXM增加关闭4*/
        | [enHeatLvlSts.EN_HEAT_LVL_1 != Tbox_Message ...
        | && enHeatLvlSts.EN_HEAT_LVL_2 != Tbox_Message ...
        | && enHeatLvlSts.EN_HEAT_LVL_3 != Tbox_Message ...
        | && 4 != Tbox_Message]
  state MessageConflictDeal [parallel]
    settings: executionOrder=3
    state Default
      en,du:
      OutMsgHMI = HMI_Message;
      OutMsgTbox = Tbox_Message;
      MixConflictFlg = FALSE;
    state VentilateConflict
      en:
      OutMsgHMI = 0;
      OutMsgTbox = 0;
      MixConflictFlg = TRUE;
    state HeatConflict
      en:
      OutMsgHMI = 0;
      OutMsgTbox = 0;
      MixConflictFlg = FALSE;
    (default) -> MessageConflictDeal.Default
    MessageConflictDeal.Default -> VentilateConflict [order 2] : /*通风加热报文同时有效 不包含关闭 */
        | [FALSE != VentValidFlag ...
        | && ((FALSE != HMI_Flag && 4 != HMI_Message)...
        | || (FALSE != Tbox_Flag && 4 != Tbox_Message))]
    VentilateConflict -> MessageConflictDeal.Default [order 2] : /*通风加热报文不同时有效或关闭，20240507NXM修改跳转顺序*/
        | [FALSE == VentValidFlag ...
        | || 4 == HMI_Message ...
        | || 4 == Tbox_Message]
    MessageConflictDeal.Default -> HeatConflict [order 1] : /*P20车型HMI、TBOX加热报文同时有效*/
        | [enProjectType.EN_PROJECT_P20 == CarTypeCfg ...
        | && FALSE != HMI_Flag ...
        | && FALSE != Tbox_Flag]
    HeatConflict -> MessageConflictDeal.Default [order 2] : /*非P20车型||P20车型加热报文不同时有效，20240507NXM*/
        | [enProjectType.EN_PROJECT_P20 != CarTypeCfg ...
        | || (enProjectType.EN_PROJECT_P20 == CarTypeCfg ...
        | && (FALSE == HMI_Flag || FALSE == Tbox_Flag))]
    VentilateConflict -> HeatConflict [order 1] : /*P20车型HMI、TBOX加热报文同时有效*/
        | [enProjectType.EN_PROJECT_P20 == CarTypeCfg ...
        | && FALSE != HMI_Flag ...
        | && FALSE != Tbox_Flag ...
        | && FALSE == VentValidFlag]
    HeatConflict -> VentilateConflict [order 1] : /*通风加热报文同时有效，20240507NXM*/
        | [FALSE != VentValidFlag ...
        | && (FALSE != HMI_Flag ...
        | || FALSE != Tbox_Flag)]
  data: CarTypeCfg input uint8; HMI_Message input; Tbox_Message input; VentValidFlag input uint8; FALSE parameter; OutMsgHMI output uint8; OutMsgTbox output uint8; HMI_Flag local uint8; Tbox_Flag local uint8; TRUE parameter; MixConflictFlg output uint8

== stateflow chart Appl_HeatAdj_CtrlModel/UpDataInputInfo/InputSignalProcess/HeatMessage/HeatMessage/MsgConflictFunction2/Function ==
  state HMI_MessageDeal [parallel]
    settings: executionOrder=1
    state Default
      en:
      HMI_Flag = FALSE;
    state Valid
      en:
      HMI_Flag = TRUE;
    (default) -> HMI_MessageDeal.Default
    HMI_MessageDeal.Default -> HMI_MessageDeal.Valid : /*HMI加热报文有效0x0:Inactive；0x1:Level 1；1档;0x2:Level 2；2档;0x3:Level 3；3档；0x4:OFF: 0x05 OPEN*/
        | [enHeatLvlSts.EN_HEAT_LVL_1 == HMI_Message ...
        | || enHeatLvlSts.EN_HEAT_LVL_2 == HMI_Message ...
        | || enHeatLvlSts.EN_HEAT_LVL_3 == HMI_Message ...
        | || 4 == HMI_Message || 5 == HMI_Message]
    HMI_MessageDeal.Valid -> HMI_MessageDeal.Default : /*HMI加热报文无效，20240507NXM增加关闭4*/
        | [enHeatLvlSts.EN_HEAT_LVL_1 != HMI_Message ...
        | && enHeatLvlSts.EN_HEAT_LVL_2 != HMI_Message ...
        | && enHeatLvlSts.EN_HEAT_LVL_3 != HMI_Message ...
        | && 4 != HMI_Message && 5 != HMI_Message]
  state Tbox_MessageDeal [parallel]
    settings: executionOrder=2
    state Default
      en:
      Tbox_Flag = FALSE;
    state Valid
      en:
      Tbox_Flag = TRUE;
    (default) -> Tbox_MessageDeal.Default
    Tbox_MessageDeal.Default -> Tbox_MessageDeal.Valid : /*Tbox加热报文有效0x0:No Request；0x1:Heat_1；0x2:Heat_2；0x3:Heat_3；0x4:Close*/
        | [enHeatLvlSts.EN_HEAT_LVL_1 == Tbox_Message ...
        | || enHeatLvlSts.EN_HEAT_LVL_2 == Tbox_Message ...
        | || enHeatLvlSts.EN_HEAT_LVL_3 == Tbox_Message ...
        | || 4 == Tbox_Message]
    Tbox_MessageDeal.Valid -> Tbox_MessageDeal.Default : /*Tbox加热报文无效，20240507NXM增加关闭4*/
        | [enHeatLvlSts.EN_HEAT_LVL_1 != Tbox_Message ...
        | && enHeatLvlSts.EN_HEAT_LVL_2 != Tbox_Message ...
        | && enHeatLvlSts.EN_HEAT_LVL_3 != Tbox_Message ...
        | && 4 != Tbox_Message]
  state MessageConflictDeal [parallel]
    settings: executionOrder=3
    state Default
      en,du:
      OutMsgHMI = HMI_Message;
      OutMsgTbox = Tbox_Message;
      MixConflictFlg = FALSE;
    state VentilateConflict
      en:
      OutMsgHMI = 0;
      OutMsgTbox = 0;
      MixConflictFlg = TRUE;
    state HeatConflict
      en:
      OutMsgHMI = 0;
      OutMsgTbox = 0;
      MixConflictFlg = FALSE;
    (default) -> MessageConflictDeal.Default
    MessageConflictDeal.Default -> VentilateConflict [order 2] : /*通风加热报文同时有效 不包含关闭 */
        | [FALSE != VentValidFlag ...
        | && ((FALSE != HMI_Flag && 4 != HMI_Message)...
        | || (FALSE != Tbox_Flag && 4 != Tbox_Message))]
    VentilateConflict -> MessageConflictDeal.Default [order 2] : /*通风加热报文不同时有效或关闭，20240507NXM修改跳转顺序*/
        | [FALSE == VentValidFlag ...
        | || 4 == HMI_Message ...
        | || 4 == Tbox_Message]
    MessageConflictDeal.Default -> HeatConflict [order 1] : /*P20车型HMI、TBOX加热报文同时有效*/
        | [enProjectType.EN_PROJECT_P20 == CarTypeCfg ...
        | && FALSE != HMI_Flag ...
        | && FALSE != Tbox_Flag]
    HeatConflict -> MessageConflictDeal.Default [order 2] : /*非P20车型||P20车型加热报文不同时有效，20240507NXM*/
        | [enProjectType.EN_PROJECT_P20 != CarTypeCfg ...
        | || (enProjectType.EN_PROJECT_P20 == CarTypeCfg ...
        | && (FALSE == HMI_Flag || FALSE == Tbox_Flag))]
    VentilateConflict -> HeatConflict [order 1] : /*P20车型HMI、TBOX加热报文同时有效*/
        | [enProjectType.EN_PROJECT_P20 == CarTypeCfg ...
        | && FALSE != HMI_Flag ...
        | && FALSE != Tbox_Flag ...
        | && FALSE == VentValidFlag]
    HeatConflict -> VentilateConflict [order 1] : /*通风加热报文同时有效，20240507NXM*/
        | [FALSE != VentValidFlag ...
        | && (FALSE != HMI_Flag ...
        | || FALSE != Tbox_Flag)]
  data: CarTypeCfg input uint8; HMI_Message input; Tbox_Message input; VentValidFlag input uint8; FALSE parameter; OutMsgHMI output uint8; OutMsgTbox output uint8; HMI_Flag local uint8; Tbox_Flag local uint8; TRUE parameter; MixConflictFlg output uint8

== stateflow chart Appl_HeatAdj_CtrlModel/LogicCtrl/LocalAdjustCtrl/HeatLevelDeal/SwLevelAquireFunction1/SwLevelAquireFunction ==
  state LevelAquire
    (default) -> (junction 181)
    LevelAquire -> (junction 181)
    (junction 181) -> (junction 177) [order 1] : /*存在禁能条件时，不再输出有效加热请求*/
        | /*加热功能禁能
        | || 通用前置条件不满足)*/
        | [enHeatStopReason.EN_HEAT_STOP_R_NONE != DisableSts ...
        | || FALSE == EnableCfg ...
        | || TRUE != ComPCFlag]
    (junction 181) -> (junction 184) [order 2] : {StopFlag = FALSE;}
    (junction 177) -> (junction 176) : {Level = enHeatLvlSts.EN_HEAT_LVL_OFF;
        | StopFlag = TRUE;}
    (junction 176) -> (junction 184)
    (junction 184) -> (junction 185)
    (junction 185) -> (junction 48) [order 1] : [FALSE == StopFlag]
    (junction 48) -> (junction 50) [order 1] : /*P20
        | 0x0:无动作
        | 0x1:开始
        | 0x2:关闭
        | 0x3:无效值*/
        | [0x02 == CAN_Message]
    (junction 185) -> (junction 188) [order 2] : {Level = enHeatLvlSts.EN_HEAT_LVL_OFF;}
    (junction 48) -> (junction 142) [order 2]
    (junction 50) -> (junction 52) : {Level = enHeatLvlSts.EN_HEAT_LVL_OFF;}
    (junction 142) -> (junction 144) [order 1] : /*P20
        | 0x0:无动作
        | 0x1:开始
        | 0x2:关闭
        | 0x3:无效值*/
        | [0x01 == CAN_Message]
    (junction 142) -> (junction 55) [order 2] : {Level = 0xFF;}
    (junction 144) -> (junction 146) : {Level = enHeatLvlSts.EN_HEAT_LVL_3;}
    (junction 55) -> (junction 188)
    (junction 146) -> (junction 55)
    (junction 52) -> (junction 146)
    (junction 188) -> (junction 75)
  data: EnableCfg input uint8; CAN_Message input uint8; DisableSts input Enum: enHeatStopReason; Level output uint8; TRUE parameter; FALSE parameter; ComPCFlag input; StopFlag local boolean

== stateflow chart Appl_HeatAdj_CtrlModel/LogicCtrl/LocalAdjustCtrl/OutputDeal/HeatOutFunction2/HeatOut/TimeDiffTs/Chart ==
  (default) -> (junction 3)
  (junction 3) -> (junction 5)
  (junction 5) -> (junction 7) [order 1] : /* 入参比当前大 */
      | [lastTs > Ts]
  (junction 5) -> (junction 13) [order 2] : {OutTs = Ts - lastTs;}
  (junction 7) -> (junction 11) : {OutTs = 0xFFFFFFFF - lastTs + Ts +1;}
  (junction 11) -> (junction 13)
  (junction 13) -> (junction 17)
  data: lastTs input uint32; Ts input uint32; OutTs output uint32

== stateflow chart Appl_HeatAdj_CtrlModel/UpDataInputInfo/InputSignalProcess/EorrorProcess/EorrorProcess/ErrorFunction3/OppositeMessageDeal ==
  state Default
    en:
    HeatErr = FALSE;
  state Fault
    en:
    HeatErr = TRUE;
  (default) -> Default
  Default -> Fault : /*任一故障输入*/
      | [FALSE != FirstFaultSts ...
      | || FALSE != SecondFaultSts]
  Fault -> Default : /*无故障输入*/
      | [FALSE == FirstFaultSts ...
      | && FALSE == SecondFaultSts]
  data: TRUE parameter; FALSE parameter; FirstFaultSts input uint8; SecondFaultSts input uint8; HeatErr output uint8

== stateflow chart Appl_HeatAdj_CtrlModel/UpDataInputInfo/InputSignalProcess/EorrorProcess/EorrorProcess/ErrorFunction4/OppositeMessageDeal ==
  state Default
    en:
    HeatErr = FALSE;
  state Fault
    en:
    HeatErr = TRUE;
  (default) -> Default
  Default -> Fault : /*任一故障输入*/
      | [FALSE != FirstFaultSts ...
      | || FALSE != SecondFaultSts]
  Fault -> Default : /*无故障输入*/
      | [FALSE == FirstFaultSts ...
      | && FALSE == SecondFaultSts]
  data: TRUE parameter; FALSE parameter; FirstFaultSts input uint8; SecondFaultSts input uint8; HeatErr output uint8

== stateflow chart Appl_HeatAdj_CtrlModel/UpDataInputInfo/InputSignalProcess/EorrorProcess/EorrorProcess/ErrorFunction5/OppositeMessageDeal ==
  state Default
    en:
    HeatErr = FALSE;
  state Fault
    en:
    HeatErr = TRUE;
  (default) -> Default
  Default -> Fault : /*任一故障输入*/
      | [FALSE != FirstFaultSts ...
      | || FALSE != SecondFaultSts]
  Fault -> Default : /*无故障输入*/
      | [FALSE == FirstFaultSts ...
      | && FALSE == SecondFaultSts]
  data: TRUE parameter; FALSE parameter; FirstFaultSts input uint8; SecondFaultSts input uint8; HeatErr output uint8

== stateflow chart Appl_HeatAdj_CtrlModel/LogicCtrl/LocalAdjustCtrl/OutputDeal/TempFunction1/TempFunction ==
  state Ts = D_HAL_GET_CUR_MS_TS [function]
  state OutTs = TimeDiffTs(lastTs,Ts) [function]
  state TempLvl
    (default) -> (junction 39)
    TempLvl -> (junction 39)
    (junction 39) -> (junction 41) [order 1] : /* P20方向盘加热等级 */
        | [enProjectType.EN_PROJECT_P20 == ProjectType ...
        | && TRUE == ThirdHeat]
    (junction 39) -> (junction 6) [order 2]
    (junction 41) -> (junction 43) : {AimTemp = D_SwsLevel_Temp;
        | TimeCnt = D_HAL_GET_CUR_MS_TS();}
    (junction 6) -> (junction 8) [order 1] : /* 等级1 */
        | [enHeatLvlSts.EN_HEAT_LVL_1 == AimLevel]
    (junction 6) -> (junction 10) [order 2]
    (junction 8) -> (junction 24) : {AimTemp = D_1stLevel_36;
        | TimeCnt = D_HAL_GET_CUR_MS_TS();}
    (junction 10) -> (junction 12) [order 1] : /* 等级2 */
        | [enHeatLvlSts.EN_HEAT_LVL_2 == AimLevel]
    (junction 10) -> (junction 14) [order 2]
    (junction 12) -> (junction 22) : {AimTemp = D_2ndLevel_39;
        | TimeCnt = D_HAL_GET_CUR_MS_TS();}
    (junction 14) -> (junction 16) [order 1] : /* 等级3 */
        | [enHeatLvlSts.EN_HEAT_LVL_3 == AimLevel]
    (junction 14) -> (junction 18) [order 2] : {AimTemp = 0;
        | TimeCnt = D_HAL_GET_CUR_MS_TS();}
    (junction 16) -> (junction 49)
    (junction 49) -> (junction 50) [order 1] : /* 小于13min 且为P20 且本次未降至 45度(防止32bit计数超时重新小于13min) */
        | [enProjectType.EN_PROJECT_P20 == ProjectType ...
        | && TimeDiffTs(TimeCnt,D_HAL_GET_CUR_MS_TS()) <= CAL_LEVEL3_TIMEOUT ...
        | && AimTemp != D_3rdLevel_45]
    (junction 49) -> (junction 20) [order 2] : {AimTemp = D_3rdLevel_45;}
    (junction 50) -> (junction 52) : {AimTemp = D_3rdLevel_48;}
    (junction 20) -> (junction 18)
    (junction 52) -> (junction 20)
    (junction 22) -> (junction 52)
    (junction 24) -> (junction 22)
    (junction 43) -> (junction 24)
    (junction 18) -> (junction 29)
  (default) -> TempLvl
  data: Ts function_output; lastTs function_input; Ts function_input; OutTs function_output; AimTemp output uint16; D_1stLevel_36 parameter; D_2ndLevel_39 parameter; AimLevel input Enum: enHeatLvlSts; ProjectType input uint8; ThirdHeat input uint8; D_SwsLevel_Temp parameter; TRUE parameter; TimeCnt local uint32; CAL_LEVEL3_TIMEOUT parameter; D_3rdLevel_45 parameter; D_3rdLevel_48 parameter

== stateflow chart Appl_HeatAdj_CtrlModel/LogicCtrl/LocalAdjustCtrl/OutputDeal/TempFunction1/TempFunction/TimeDiffTs/Chart ==
  (default) -> (junction 3)
  (junction 3) -> (junction 5)
  (junction 5) -> (junction 7) [order 1] : /* 入参比当前大 */
      | [lastTs > Ts]
  (junction 5) -> (junction 13) [order 2] : {OutTs = Ts - lastTs;}
  (junction 7) -> (junction 11) : {OutTs = 0xFFFFFFFF - lastTs + Ts +1;}
  (junction 11) -> (junction 13)
  (junction 13) -> (junction 17)
  data: lastTs input uint32; Ts input uint32; OutTs output uint32

== stateflow chart Appl_HeatAdj_CtrlModel/LogicCtrl/LocalAdjustCtrl/OutputDeal/TempFunction/TempFunction/TimeDiffTs/Chart ==
  (default) -> (junction 3)
  (junction 3) -> (junction 5)
  (junction 5) -> (junction 7) [order 1] : /* 入参比当前大 */
      | [lastTs > Ts]
  (junction 5) -> (junction 13) [order 2] : {OutTs = Ts - lastTs;}
  (junction 7) -> (junction 11) : {OutTs = 0xFFFFFFFF - lastTs + Ts +1;}
  (junction 11) -> (junction 13)
  (junction 13) -> (junction 17)
  data: lastTs input uint32; Ts input uint32; OutTs output uint32
